simulink library "dkc"  (R2021b)
settings: Solver=VariableStepAuto  StartTime=0.0  StopTime=10.0  RelTol=1e-3
undefined symbols (not defined in the file or in its folder): ENUM_ANTITHEFT_ALARM, ENUM_ANTITHEFT_ARM, ENUM_ANTITHEFT_DISARM, ENUM_ANTITHEFT_WAIT, ENUM_BTCONNSTA_CONNECTED, ENUM_BTConnSta_CONNECTED, ENUM_BTCONNSTA_DISCONNECTED, ENUM_DKCAuthSta_DECRYPTIONFAIL, ENUM_DKCAuthSta_NORMAL, ENUM_DKCAuthSta_TIMEERROR, ENUM_DKCPCMDHANDING_FORCELIFT, ENUM_DKCPCMDHANDING_LOCK, ENUM_DKCPCMDHANDING_LOCKTGATEFAIL, ENUM_DKCPCMDHANDING_OVER, ENUM_DKCPCMDHANDING_TGATEHANDLE, ENUM_DKCPCMDHANDING_UNLOCK, ENUM_DkeyShowIVI_DEFAULT, ENUM_DkeyShowIVI_INVALID, ENUM_DkeyShowIVI_NFCGREEN, ENUM_DkeyShowIVI_NFCRED, ENUM_GEARACTUALPOSN_N, ENUM_GEARACTUALPOSN_P, ENUM_KEYMISSSTA_DEFAULT, ENUM_KEYMISSSTA_KEYMISS, ENUM_KEYMODE_DAFAULT, ENUM_KEYMODE_INVALID, ENUM_KEYMODE_NFC, ENUM_KEYMODE_UIDBLE, ENUM_KEYMODE_UIDUWB, ENUM_KEYTYPE_NFC, ENUM_KEYTYPE_NOREQ, ENUM_KEYTYPE_UID, ENUM_PCMDTOBCM_DEFAULT, ENUM_PCMDTOBCM_FORCELIFT, ENUM_PCMDTOBCM_LOCK, ENUM_PCMDTOBCM_LOCKTGATEFAIL, ENUM_PCMDTOBCM_NFCCOMMAND, ENUM_PCMDTOBCM_REMOTETGATE, ENUM_PCMDTOBCM_TGATEHANDLE, ENUM_PCMDTOBCM_UNLOCK, ENUM_PCMDTOBCM_UWBLOCK, ENUM_PCMDTOBCM_UWBUNLOCK, ENUM_PDKEYPTGRAW_INTOZONE, ENUM_PDKEYPTGRAW_OUTZONE, ENUM_PDKEYPTGRAW_UNAVALIABLE, ENUM_PDKEYRAWLULOCK_INLOCK, ENUM_PDKEYRAWLULOCK_INUNLOCK, ENUM_PDKEYRAWLULOCK_UNAVALIABLE, ENUM_PDKEYRAWPS_INPS, ENUM_PDKEYRAWPS_OUTPS, ENUM_PDKEYRAWPS_UNAVALIABLE, ENUM_PDKEYSPTGRAW_INTOZONE, ENUM_PDKEYSPTGRAW_OUTZONE, ENUM_PDKEYSPTGRAW_UNAVALIABLE, ENUM_PDKEYWELCOMERAW_INTOZONE, ENUM_PDKEYWELCOMERAW_UNAVALIABLE, ENUM_POWERSTA_OFF, ENUM_POWERSTA_OFFA, ENUM_POWERSTA_OFFC, ENUM_POWERSTA_ON ... (+79)
libraries: simulink x99, hcu_lib x6
(part 3 of 4)

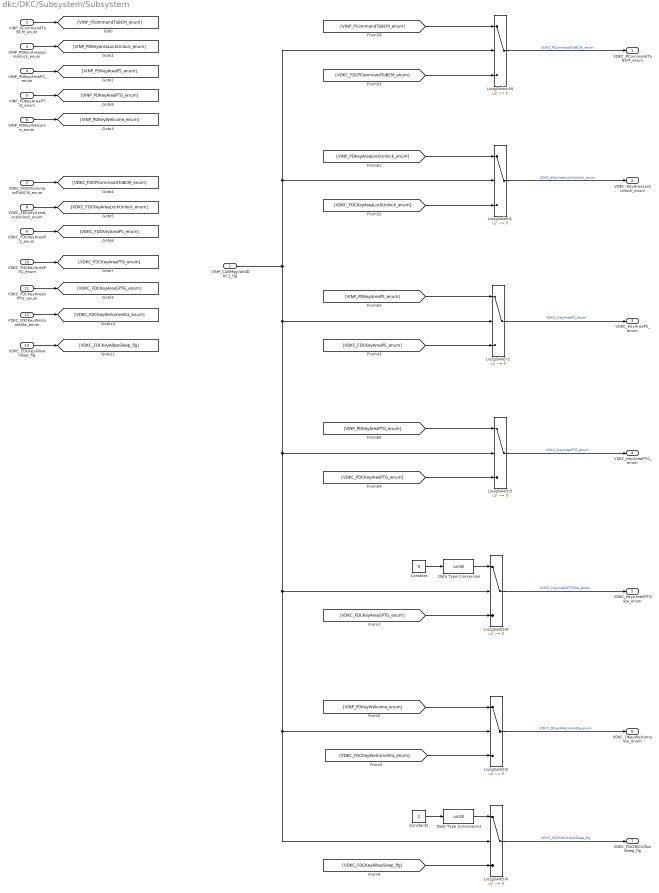
== system dkc/DKC/Subsystem/Subsystem ==
  VINP_CANMsgValidDKC1_flg : Inport
  VINP_PCommandToBCM_enum : Inport  Port=2
  VINP_PDKeyAreaLockUnlock_enum : Inport  Port=3
  VINP_PDKeyAreaPS_enum : Inport  Port=4
  VINP_PDKeyAreaPTG_enum : Inport  Port=5
  VINP_PDKeyWelcome_enum : Inport  Port=6
  VDKC_FDCPCommandToBCM_enum : Inport  Port=7
  VDKC_FDCKeyAreaLockUnlock_enum : Inport  Port=8
  VDKC_FDCKeyAreaPS_enum : Inport  Port=9
  VDKC_FDCKeyAreaPTG_enum : Inport  Port=10
  VDKC_FDCKeyAreaSPTG_enum : Inport  Port=11
  VDKC_FDCKeyWelcomeSta_enum : Inport  Port=12
  VDKC_FDCKeyAllowSleep_flg : Inport  Port=13
  Constant : Constant  Value=0
  Constant1 : Constant
  Data Type Conversion : DataTypeConversion  OutDataTypeStr=uint8
  Data Type Conversion1 : DataTypeConversion  OutDataTypeStr=uint8
  LiuzgSwitch{1..6,16} (7 alike) : Switch  Criteria=u2 ~= 0
      settings: AttributesFormatString=<%<Criteria>>
  VDKC_PCommandToBCM_enum : Outport
  VDKC_KeyAreaLockUnlock_enum : Outport  Port=2
  VDKC_KeyAreaPS_enum : Outport  Port=3
  VDKC_KeyAreaPTG_enum : Outport  Port=4
  VDKC_KeyAreaSPTGSta_enum : Outport  Port=5
  VDKC_DKeyWelcomeSta_enum : Outport  Port=6
  VDKC_FDCDKCAllowSleep_flg : Outport  Port=7
  wires:
  LiuzgSwitch6/1 -> VDKC_FDCDKCAllowSleep_flg/1  "VDKC_FDCDKCAllowSleep_flg"
  [VDKC_FDCKeyAllowSleep_flg] -> LiuzgSwitch6/3
  Data Type Conversion1/1 -> LiuzgSwitch6/1
  Constant1/1 -> Data Type Conversion1/1
  VDKC_FDCKeyAllowSleep_flg/1 -> [VDKC_FDCKeyAllowSleep_flg]
  Constant/1 -> Data Type Conversion/1
  Data Type Conversion/1 -> LiuzgSwitch4/1
  [VDKC_FDCKeyAreaSPTG_enum] -> LiuzgSwitch4/3
  VDKC_FDCKeyAreaSPTG_enum/1 -> [VDKC_FDCKeyAreaSPTG_enum]
  [VINP_PDKeyAreaPTG_enum] -> LiuzgSwitch3/1
  LiuzgSwitch4/1 -> VDKC_KeyAreaSPTGSta_enum/1  "VDKC_KeyAreaSPTGSta_enum"
  VINP_CANMsgValidDKC1_flg/1 -> LiuzgSwitch1/2, LiuzgSwitch16/2, LiuzgSwitch3/2, LiuzgSwitch6/2, LiuzgSwitch5/2, LiuzgSwitch4/2, LiuzgSwitch2/2
  VINP_PDKeyAreaPTG_enum/1 -> [VINP_PDKeyAreaPTG_enum]
  [VDKC_FDCKeyAreaPS_enum] -> LiuzgSwitch2/3
  [VDKC_FDCKeyAreaPTG_enum] -> LiuzgSwitch3/3
  LiuzgSwitch2/1 -> VDKC_KeyAreaPS_enum/1  "VDKC_KeyAreaPS_enum"
  [VINP_PCommandToBCM_enum] -> LiuzgSwitch16/1
  LiuzgSwitch3/1 -> VDKC_KeyAreaPTG_enum/1  "VDKC_KeyAreaPTG_enum"
  [VINP_PDKeyAreaLockUnlock_enum] -> LiuzgSwitch1/1
  [VDKC_FDCPCommandToBCM_enum] -> LiuzgSwitch16/3
  [VDKC_FDCKeyAreaLockUnlock_enum] -> LiuzgSwitch1/3
  [VINP_PDKeyAreaPS_enum] -> LiuzgSwitch2/1
  LiuzgSwitch16/1 -> VDKC_PCommandToBCM_enum/1  "VDKC_PCommandToBCM_enum"
  LiuzgSwitch1/1 -> VDKC_KeyAreaLockUnlock_enum/1  "VDKC_KeyAreaLockUnlock_enum"
  VINP_PCommandToBCM_enum/1 -> [VINP_PCommandToBCM_enum]
  VINP_PDKeyAreaLockUnlock_enum/1 -> [VINP_PDKeyAreaLockUnlock_enum]
  VINP_PDKeyAreaPS_enum/1 -> [VINP_PDKeyAreaPS_enum]
  VDKC_FDCKeyAreaPTG_enum/1 -> [VDKC_FDCKeyAreaPTG_enum]
  VDKC_FDCKeyAreaPS_enum/1 -> [VDKC_FDCKeyAreaPS_enum]
  VDKC_FDCKeyAreaLockUnlock_enum/1 -> [VDKC_FDCKeyAreaLockUnlock_enum]
  VDKC_FDCPCommandToBCM_enum/1 -> [VDKC_FDCPCommandToBCM_enum]
  LiuzgSwitch5/1 -> VDKC_DKeyWelcomeSta_enum/1  "VDKC_DKeyWelcomeSta_enum"
  VINP_PDKeyWelcome_enum/1 -> [VINP_PDKeyWelcome_enum]
  [VINP_PDKeyWelcome_enum] -> LiuzgSwitch5/1
  VDKC_FDCKeyWelcomeSta_enum/1 -> [VDKC_FDCKeyWelcomeSta_enum]
  [VDKC_FDCKeyWelcomeSta_enum] -> LiuzgSwitch5/3

== system dkc/DKC/Subsystem/Triggered Subsystem ==
  Trigger : TriggerPort  TriggerType=function-call  VariantControl=(inherit)
  RollingCounter : Subsystem  mask{CounterMAX=4294967295}
      mask help: MeasumentTrigerEvent
      mask Display: fprintf('RollingCounter');
  DKCTimeSN : Outport
  wires:
  RollingCounter/1(out) -> DKCTimeSN/1

== system dkc/DKC/Subsystem/DKC_Handler/SR_Latch1 ==
  set : Inport
  reset : Inport  Port=2
  Data Type Conversion : DataTypeConversion  OutDataTypeStr=boolean
  Logical Operator : Logic  AllPortsSameDT=off  OutDataTypeStr=boolean
  Logical Operator1 : Logic  Operator=NOT  AllPortsSameDT=off  OutDataTypeStr=boolean
  Switch1 : Switch  Criteria=u2 ~= 0  Threshold=0.5
      settings: AttributesFormatString=<Criteria=%<Criteria>>
  Switch2 : Switch  Criteria=u2 ~= 0  Threshold=0.5
      settings: AttributesFormatString=<Criteria=%<Criteria>>
  Unit Delay : UnitDelay  SampleTime=-1  HasFrameUpgradeWarning=on
  latched : Outport
  wires:
  Logical Operator1/1 -> Switch2/1, Logical Operator/2
  Logical Operator/1 -> Switch1/2
  Switch2/1 -> Switch1/3
  Unit Delay/1 -> Switch2/3
  reset/1 -> Logical Operator1/1, Switch2/2
  set/1 -> Logical Operator/1, Switch1/1
  Switch1/1 -> Data Type Conversion/1
  Data Type Conversion/1 -> latched/1, Unit Delay/1

== system dkc/DKC/Subsystem/DKC_Handler/SR_Latch10 ==
  set : Inport
  reset : Inport  Port=2
  Data Type Conversion : DataTypeConversion  OutDataTypeStr=boolean
  Logical Operator : Logic  AllPortsSameDT=off  OutDataTypeStr=boolean
  Logical Operator1 : Logic  Operator=NOT  AllPortsSameDT=off  OutDataTypeStr=boolean
  Switch1 : Switch  Criteria=u2 ~= 0  Threshold=0.5
      settings: AttributesFormatString=<Criteria=%<Criteria>>
  Switch2 : Switch  Criteria=u2 ~= 0  Threshold=0.5
      settings: AttributesFormatString=<Criteria=%<Criteria>>
  Unit Delay : UnitDelay  SampleTime=-1  HasFrameUpgradeWarning=on
  latched : Outport
  wires:
  Logical Operator1/1 -> Switch2/1, Logical Operator/2
  Logical Operator/1 -> Switch1/2
  Switch2/1 -> Switch1/3
  Unit Delay/1 -> Switch2/3
  reset/1 -> Logical Operator1/1, Switch2/2
  set/1 -> Logical Operator/1, Switch1/1
  Switch1/1 -> Data Type Conversion/1
  Data Type Conversion/1 -> latched/1, Unit Delay/1

== system dkc/DKC/Subsystem/DKC_Handler/SR_Latch11 ==
  set : Inport
  reset : Inport  Port=2
  Data Type Conversion : DataTypeConversion  OutDataTypeStr=boolean
  Logical Operator : Logic  AllPortsSameDT=off  OutDataTypeStr=boolean
  Logical Operator1 : Logic  Operator=NOT  AllPortsSameDT=off  OutDataTypeStr=boolean
  Switch1 : Switch  Criteria=u2 ~= 0  Threshold=0.5
      settings: AttributesFormatString=<Criteria=%<Criteria>>
  Switch2 : Switch  Criteria=u2 ~= 0  Threshold=0.5
      settings: AttributesFormatString=<Criteria=%<Criteria>>
  Unit Delay : UnitDelay  SampleTime=-1  HasFrameUpgradeWarning=on
  latched : Outport
  wires:
  Data Type Conversion/1 -> Unit Delay/1, latched/1
  Switch1/1 -> Data Type Conversion/1
  set/1 -> Switch1/1, Logical Operator/1
  reset/1 -> Switch2/2, Logical Operator1/1
  Unit Delay/1 -> Switch2/3
  Switch2/1 -> Switch1/3
  Logical Operator/1 -> Switch1/2
  Logical Operator1/1 -> Logical Operator/2, Switch2/1

== system dkc/DKC/Subsystem/DKC_Handler/SR_Latch12 ==
  set : Inport
  reset : Inport  Port=2
  Data Type Conversion : DataTypeConversion  OutDataTypeStr=boolean
  Logical Operator : Logic  AllPortsSameDT=off  OutDataTypeStr=boolean
  Logical Operator1 : Logic  Operator=NOT  AllPortsSameDT=off  OutDataTypeStr=boolean
  Switch1 : Switch  Criteria=u2 ~= 0  Threshold=0.5
      settings: AttributesFormatString=<Criteria=%<Criteria>>
  Switch2 : Switch  Criteria=u2 ~= 0  Threshold=0.5
      settings: AttributesFormatString=<Criteria=%<Criteria>>
  Unit Delay : UnitDelay  SampleTime=-1  HasFrameUpgradeWarning=on
  latched : Outport
  wires:
  Data Type Conversion/1 -> Unit Delay/1, latched/1
  Switch1/1 -> Data Type Conversion/1
  set/1 -> Switch1/1, Logical Operator/1
  reset/1 -> Switch2/2, Logical Operator1/1
  Unit Delay/1 -> Switch2/3
  Switch2/1 -> Switch1/3
  Logical Operator/1 -> Switch1/2
  Logical Operator1/1 -> Logical Operator/2, Switch2/1

== system dkc/DKC/Subsystem/DKC_Handler/SR_Latch13 ==
  set : Inport
  reset : Inport  Port=2
  Data Type Conversion : DataTypeConversion  OutDataTypeStr=boolean
  Logical Operator : Logic  AllPortsSameDT=off  OutDataTypeStr=boolean
  Logical Operator1 : Logic  Operator=NOT  AllPortsSameDT=off  OutDataTypeStr=boolean
  Switch1 : Switch  Criteria=u2 ~= 0  Threshold=0.5
      settings: AttributesFormatString=<Criteria=%<Criteria>>
  Switch2 : Switch  Criteria=u2 ~= 0  Threshold=0.5
      settings: AttributesFormatString=<Criteria=%<Criteria>>
  Unit Delay : UnitDelay  SampleTime=-1  HasFrameUpgradeWarning=on
  latched : Outport
  wires:
  Logical Operator1/1 -> Switch2/1, Logical Operator/2
  Logical Operator/1 -> Switch1/2
  Switch2/1 -> Switch1/3
  Unit Delay/1 -> Switch2/3
  reset/1 -> Logical Operator1/1, Switch2/2
  set/1 -> Logical Operator/1, Switch1/1
  Switch1/1 -> Data Type Conversion/1
  Data Type Conversion/1 -> latched/1, Unit Delay/1

== system dkc/DKC/Subsystem/DKC_Handler/SR_Latch14 ==
  set : Inport
  reset : Inport  Port=2
  Data Type Conversion : DataTypeConversion  OutDataTypeStr=boolean
  Logical Operator : Logic  AllPortsSameDT=off  OutDataTypeStr=boolean
  Logical Operator1 : Logic  Operator=NOT  AllPortsSameDT=off  OutDataTypeStr=boolean
  Switch1 : Switch  Criteria=u2 ~= 0  Threshold=0.5
      settings: AttributesFormatString=<Criteria=%<Criteria>>
  Switch2 : Switch  Criteria=u2 ~= 0  Threshold=0.5
      settings: AttributesFormatString=<Criteria=%<Criteria>>
  Unit Delay : UnitDelay  SampleTime=-1  HasFrameUpgradeWarning=on
  latched : Outport
  wires:
  Data Type Conversion/1 -> Unit Delay/1, latched/1
  Switch1/1 -> Data Type Conversion/1
  set/1 -> Switch1/1, Logical Operator/1
  reset/1 -> Switch2/2, Logical Operator1/1
  Unit Delay/1 -> Switch2/3
  Switch2/1 -> Switch1/3
  Logical Operator/1 -> Switch1/2
  Logical Operator1/1 -> Logical Operator/2, Switch2/1

== system dkc/DKC/Subsystem/DKC_Handler/SR_Latch15 ==
  set : Inport
  reset : Inport  Port=2
  Data Type Conversion : DataTypeConversion  OutDataTypeStr=boolean
  Logical Operator : Logic  AllPortsSameDT=off  OutDataTypeStr=boolean
  Logical Operator1 : Logic  Operator=NOT  AllPortsSameDT=off  OutDataTypeStr=boolean
  Switch1 : Switch  Criteria=u2 ~= 0  Threshold=0.5
      settings: AttributesFormatString=<Criteria=%<Criteria>>
  Switch2 : Switch  Criteria=u2 ~= 0  Threshold=0.5
      settings: AttributesFormatString=<Criteria=%<Criteria>>
  Unit Delay : UnitDelay  SampleTime=-1  HasFrameUpgradeWarning=on
  latched : Outport
  wires:
  Logical Operator1/1 -> Switch2/1, Logical Operator/2
  Logical Operator/1 -> Switch1/2
  Switch2/1 -> Switch1/3
  Unit Delay/1 -> Switch2/3
  reset/1 -> Logical Operator1/1, Switch2/2
  set/1 -> Logical Operator/1, Switch1/1
  Switch1/1 -> Data Type Conversion/1
  Data Type Conversion/1 -> latched/1, Unit Delay/1

== system dkc/DKC/Subsystem/DKC_Handler/SR_Latch16 ==
  set : Inport
  reset : Inport  Port=2
  Data Type Conversion : DataTypeConversion  OutDataTypeStr=boolean
  Logical Operator : Logic  AllPortsSameDT=off  OutDataTypeStr=boolean
  Logical Operator1 : Logic  Operator=NOT  AllPortsSameDT=off  OutDataTypeStr=boolean
  Switch1 : Switch  Criteria=u2 ~= 0  Threshold=0.5
      settings: AttributesFormatString=<Criteria=%<Criteria>>
  Switch2 : Switch  Criteria=u2 ~= 0  Threshold=0.5
      settings: AttributesFormatString=<Criteria=%<Criteria>>
  Unit Delay : UnitDelay  SampleTime=-1  HasFrameUpgradeWarning=on
  latched : Outport
  wires:
  Data Type Conversion/1 -> Unit Delay/1, latched/1
  Switch1/1 -> Data Type Conversion/1
  set/1 -> Switch1/1, Logical Operator/1
  reset/1 -> Switch2/2, Logical Operator1/1
  Unit Delay/1 -> Switch2/3
  Switch2/1 -> Switch1/3
  Logical Operator/1 -> Switch1/2
  Logical Operator1/1 -> Logical Operator/2, Switch2/1

== system dkc/DKC/Subsystem/DKC_Handler/SR_Latch17 ==
  set : Inport
  reset : Inport  Port=2
  Data Type Conversion : DataTypeConversion  OutDataTypeStr=boolean
  Logical Operator : Logic  AllPortsSameDT=off  OutDataTypeStr=boolean
  Logical Operator1 : Logic  Operator=NOT  AllPortsSameDT=off  OutDataTypeStr=boolean
  Switch1 : Switch  Criteria=u2 ~= 0  Threshold=0.5
      settings: AttributesFormatString=<Criteria=%<Criteria>>
  Switch2 : Switch  Criteria=u2 ~= 0  Threshold=0.5
      settings: AttributesFormatString=<Criteria=%<Criteria>>
  Unit Delay : UnitDelay  SampleTime=-1  HasFrameUpgradeWarning=on
  latched : Outport
  wires:
  Logical Operator1/1 -> Switch2/1, Logical Operator/2
  Logical Operator/1 -> Switch1/2
  Switch2/1 -> Switch1/3
  Unit Delay/1 -> Switch2/3
  reset/1 -> Logical Operator1/1, Switch2/2
  set/1 -> Logical Operator/1, Switch1/1
  Switch1/1 -> Data Type Conversion/1
  Data Type Conversion/1 -> latched/1, Unit Delay/1

== system dkc/DKC/Subsystem/DKC_Handler/SR_Latch18 ==
  set : Inport
  reset : Inport  Port=2
  Data Type Conversion : DataTypeConversion  OutDataTypeStr=boolean
  Logical Operator : Logic  AllPortsSameDT=off  OutDataTypeStr=boolean
  Logical Operator1 : Logic  Operator=NOT  AllPortsSameDT=off  OutDataTypeStr=boolean
  Switch1 : Switch  Criteria=u2 ~= 0  Threshold=0.5
      settings: AttributesFormatString=<Criteria=%<Criteria>>
  Switch2 : Switch  Criteria=u2 ~= 0  Threshold=0.5
      settings: AttributesFormatString=<Criteria=%<Criteria>>
  Unit Delay : UnitDelay  SampleTime=-1  HasFrameUpgradeWarning=on
  latched : Outport
  wires:
  Data Type Conversion/1 -> Unit Delay/1, latched/1
  Switch1/1 -> Data Type Conversion/1
  set/1 -> Switch1/1, Logical Operator/1
  reset/1 -> Switch2/2, Logical Operator1/1
  Unit Delay/1 -> Switch2/3
  Switch2/1 -> Switch1/3
  Logical Operator/1 -> Switch1/2
  Logical Operator1/1 -> Logical Operator/2, Switch2/1

== system dkc/DKC/Subsystem/DKC_Handler/SR_Latch19 ==
  set : Inport
  reset : Inport  Port=2
  Data Type Conversion : DataTypeConversion  OutDataTypeStr=boolean
  Logical Operator : Logic  AllPortsSameDT=off  OutDataTypeStr=boolean
  Logical Operator1 : Logic  Operator=NOT  AllPortsSameDT=off  OutDataTypeStr=boolean
  Switch1 : Switch  Criteria=u2 ~= 0  Threshold=0.5
      settings: AttributesFormatString=<Criteria=%<Criteria>>
  Switch2 : Switch  Criteria=u2 ~= 0  Threshold=0.5
      settings: AttributesFormatString=<Criteria=%<Criteria>>
  Unit Delay : UnitDelay  SampleTime=-1  HasFrameUpgradeWarning=on
  latched : Outport
  wires:
  Data Type Conversion/1 -> Unit Delay/1, latched/1
  Switch1/1 -> Data Type Conversion/1
  set/1 -> Switch1/1, Logical Operator/1
  reset/1 -> Switch2/2, Logical Operator1/1
  Unit Delay/1 -> Switch2/3
  Switch2/1 -> Switch1/3
  Logical Operator/1 -> Switch1/2
  Logical Operator1/1 -> Logical Operator/2, Switch2/1

== system dkc/DKC/Subsystem/DKC_Handler/SR_Latch2 ==
  set : Inport
  reset : Inport  Port=2
  Data Type Conversion : DataTypeConversion  OutDataTypeStr=boolean
  Logical Operator : Logic  AllPortsSameDT=off  OutDataTypeStr=boolean
  Logical Operator1 : Logic  Operator=NOT  AllPortsSameDT=off  OutDataTypeStr=boolean
  Switch1 : Switch  Criteria=u2 ~= 0  Threshold=0.5
      settings: AttributesFormatString=<Criteria=%<Criteria>>
  Switch2 : Switch  Criteria=u2 ~= 0  Threshold=0.5
      settings: AttributesFormatString=<Criteria=%<Criteria>>
  Unit Delay : UnitDelay  SampleTime=-1  HasFrameUpgradeWarning=on
  latched : Outport
  wires:
  Data Type Conversion/1 -> Unit Delay/1, latched/1
  Switch1/1 -> Data Type Conversion/1
  set/1 -> Switch1/1, Logical Operator/1
  reset/1 -> Switch2/2, Logical Operator1/1
  Unit Delay/1 -> Switch2/3
  Switch2/1 -> Switch1/3
  Logical Operator/1 -> Switch1/2
  Logical Operator1/1 -> Logical Operator/2, Switch2/1

== system dkc/DKC/Subsystem/DKC_Handler/SR_Latch20 ==
  set : Inport
  reset : Inport  Port=2
  Data Type Conversion : DataTypeConversion  OutDataTypeStr=boolean
  Logical Operator : Logic  AllPortsSameDT=off  OutDataTypeStr=boolean
  Logical Operator1 : Logic  Operator=NOT  AllPortsSameDT=off  OutDataTypeStr=boolean
  Switch1 : Switch  Criteria=u2 ~= 0  Threshold=0.5
      settings: AttributesFormatString=<Criteria=%<Criteria>>
  Switch2 : Switch  Criteria=u2 ~= 0  Threshold=0.5
      settings: AttributesFormatString=<Criteria=%<Criteria>>
  Unit Delay : UnitDelay  SampleTime=-1  HasFrameUpgradeWarning=on
  latched : Outport
  wires:
  Data Type Conversion/1 -> Unit Delay/1, latched/1
  Switch1/1 -> Data Type Conversion/1
  set/1 -> Switch1/1, Logical Operator/1
  reset/1 -> Switch2/2, Logical Operator1/1
  Unit Delay/1 -> Switch2/3
  Switch2/1 -> Switch1/3
  Logical Operator/1 -> Switch1/2
  Logical Operator1/1 -> Logical Operator/2, Switch2/1

== system dkc/DKC/Subsystem/DKC_Handler/SR_Latch4 ==
  set : Inport
  reset : Inport  Port=2
  Data Type Conversion : DataTypeConversion  OutDataTypeStr=boolean
  Logical Operator : Logic  AllPortsSameDT=off  OutDataTypeStr=boolean
  Logical Operator1 : Logic  Operator=NOT  AllPortsSameDT=off  OutDataTypeStr=boolean
  Switch1 : Switch  Criteria=u2 ~= 0  Threshold=0.5
      settings: AttributesFormatString=<Criteria=%<Criteria>>
  Switch2 : Switch  Criteria=u2 ~= 0  Threshold=0.5
      settings: AttributesFormatString=<Criteria=%<Criteria>>
  Unit Delay : UnitDelay  SampleTime=-1  HasFrameUpgradeWarning=on
  latched : Outport
  wires:
  Logical Operator1/1 -> Switch2/1, Logical Operator/2
  Logical Operator/1 -> Switch1/2
  Switch2/1 -> Switch1/3
  Unit Delay/1 -> Switch2/3
  reset/1 -> Logical Operator1/1, Switch2/2
  set/1 -> Logical Operator/1, Switch1/1
  Switch1/1 -> Data Type Conversion/1
  Data Type Conversion/1 -> latched/1, Unit Delay/1

== system dkc/DKC/Subsystem/DKC_Handler/SR_Latch5 ==
  set : Inport
  reset : Inport  Port=2
  Data Type Conversion : DataTypeConversion  OutDataTypeStr=boolean
  Logical Operator : Logic  AllPortsSameDT=off  OutDataTypeStr=boolean
  Logical Operator1 : Logic  Operator=NOT  AllPortsSameDT=off  OutDataTypeStr=boolean
  Switch1 : Switch  Criteria=u2 ~= 0  Threshold=0.5
      settings: AttributesFormatString=<Criteria=%<Criteria>>
  Switch2 : Switch  Criteria=u2 ~= 0  Threshold=0.5
      settings: AttributesFormatString=<Criteria=%<Criteria>>
  Unit Delay : UnitDelay  SampleTime=-1  HasFrameUpgradeWarning=on
  latched : Outport
  wires:
  Data Type Conversion/1 -> Unit Delay/1, latched/1
  Switch1/1 -> Data Type Conversion/1
  set/1 -> Switch1/1, Logical Operator/1
  reset/1 -> Switch2/2, Logical Operator1/1
  Unit Delay/1 -> Switch2/3
  Switch2/1 -> Switch1/3
  Logical Operator/1 -> Switch1/2
  Logical Operator1/1 -> Logical Operator/2, Switch2/1

== system dkc/DKC/Subsystem/DKC_Handler/SR_Latch6 ==
  set : Inport
  reset : Inport  Port=2
  Data Type Conversion : DataTypeConversion  OutDataTypeStr=boolean
  Logical Operator : Logic  AllPortsSameDT=off  OutDataTypeStr=boolean
  Logical Operator1 : Logic  Operator=NOT  AllPortsSameDT=off  OutDataTypeStr=boolean
  Switch1 : Switch  Criteria=u2 ~= 0  Threshold=0.5
      settings: AttributesFormatString=<Criteria=%<Criteria>>
  Switch2 : Switch  Criteria=u2 ~= 0  Threshold=0.5
      settings: AttributesFormatString=<Criteria=%<Criteria>>
  Unit Delay : UnitDelay  SampleTime=-1  HasFrameUpgradeWarning=on
  latched : Outport
  wires:
  Logical Operator1/1 -> Switch2/1, Logical Operator/2
  Logical Operator/1 -> Switch1/2
  Switch2/1 -> Switch1/3
  Unit Delay/1 -> Switch2/3
  reset/1 -> Logical Operator1/1, Switch2/2
  set/1 -> Logical Operator/1, Switch1/1
  Switch1/1 -> Data Type Conversion/1
  Data Type Conversion/1 -> latched/1, Unit Delay/1

== system dkc/DKC/Subsystem/DKC_Handler/SR_Latch8 ==
  set : Inport
  reset : Inport  Port=2
  Data Type Conversion : DataTypeConversion  OutDataTypeStr=boolean
  Logical Operator : Logic  AllPortsSameDT=off  OutDataTypeStr=boolean
  Logical Operator1 : Logic  Operator=NOT  AllPortsSameDT=off  OutDataTypeStr=boolean
  Switch1 : Switch  Criteria=u2 ~= 0  Threshold=0.5
      settings: AttributesFormatString=<Criteria=%<Criteria>>
  Switch2 : Switch  Criteria=u2 ~= 0  Threshold=0.5
      settings: AttributesFormatString=<Criteria=%<Criteria>>
  Unit Delay : UnitDelay  SampleTime=-1  HasFrameUpgradeWarning=on
  latched : Outport
  wires:
  Logical Operator1/1 -> Switch2/1, Logical Operator/2
  Logical Operator/1 -> Switch1/2
  Switch2/1 -> Switch1/3
  Unit Delay/1 -> Switch2/3
  reset/1 -> Logical Operator1/1, Switch2/2
  set/1 -> Logical Operator/1, Switch1/1
  Switch1/1 -> Data Type Conversion/1
  Data Type Conversion/1 -> latched/1, Unit Delay/1

== system dkc/DKC/Subsystem/DKC_Handler/SR_Latch9 ==
  set : Inport
  reset : Inport  Port=2
  Data Type Conversion : DataTypeConversion  OutDataTypeStr=boolean
  Logical Operator : Logic  AllPortsSameDT=off  OutDataTypeStr=boolean
  Logical Operator1 : Logic  Operator=NOT  AllPortsSameDT=off  OutDataTypeStr=boolean
  Switch1 : Switch  Criteria=u2 ~= 0  Threshold=0.5
      settings: AttributesFormatString=<Criteria=%<Criteria>>
  Switch2 : Switch  Criteria=u2 ~= 0  Threshold=0.5
      settings: AttributesFormatString=<Criteria=%<Criteria>>
  Unit Delay : UnitDelay  SampleTime=-1  HasFrameUpgradeWarning=on
  latched : Outport
  wires:
  Data Type Conversion/1 -> Unit Delay/1, latched/1
  Switch1/1 -> Data Type Conversion/1
  set/1 -> Switch1/1, Logical Operator/1
  reset/1 -> Switch2/2, Logical Operator1/1
  Unit Delay/1 -> Switch2/3
  Switch2/1 -> Switch1/3
  Logical Operator/1 -> Switch1/2
  Logical Operator1/1 -> Logical Operator/2, Switch2/1

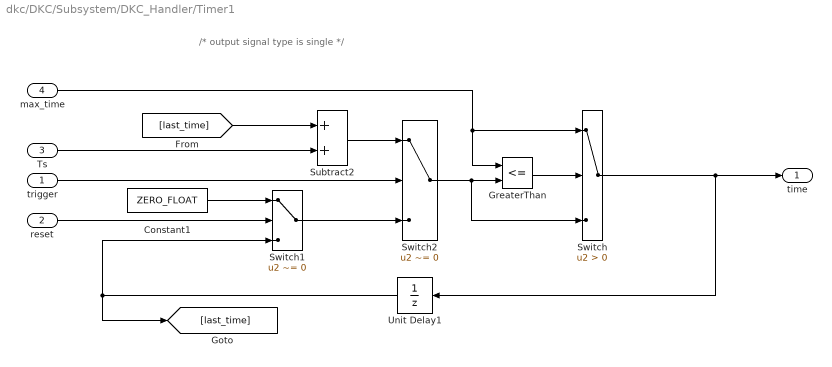
== system dkc/DKC/Subsystem/DKC_Handler/Timer1 ==
  note: /* output signal type is single */
  trigger : Inport
  reset : Inport  Port=2
  Ts : Inport  Port=3
  max_time : Inport  Port=4
  Constant1 : Constant  Value=ZERO_FLOAT  OutDataTypeStr=single
  GreaterThan : RelationalOperator  Operator=<=  OutDataTypeStr=boolean  RndMeth=Simplest
  Subtract2 : Sum
  Switch : Switch  Criteria=u2 > Threshold
  Switch1 : Switch  Criteria=u2 ~= 0
      settings: AttributesFormatString=<%<Criteria>>
  Switch2 : Switch  Criteria=u2 ~= 0
      settings: AttributesFormatString=<%<Criteria>>
  Unit Delay1 : UnitDelay  SampleTime=-1  HasFrameUpgradeWarning=on
      settings: AttributesFormatString=<initial = %<X0>>
  time : Outport
  wires:
  [last_time] -> Subtract2/1
  max_time/1 -> Switch/1, GreaterThan/1
  Unit Delay1/1 -> [last_time], Switch1/3
  Switch/1 -> time/1, Unit Delay1/1
  Switch2/1 -> Switch/3, GreaterThan/2
  Ts/1 -> Subtract2/2
  Switch1/1 -> Switch2/3
  Constant1/1 -> Switch1/1
  reset/1 -> Switch1/2
  trigger/1 -> Switch2/2
  Subtract2/1 -> Switch2/1
  GreaterThan/1 -> Switch/2

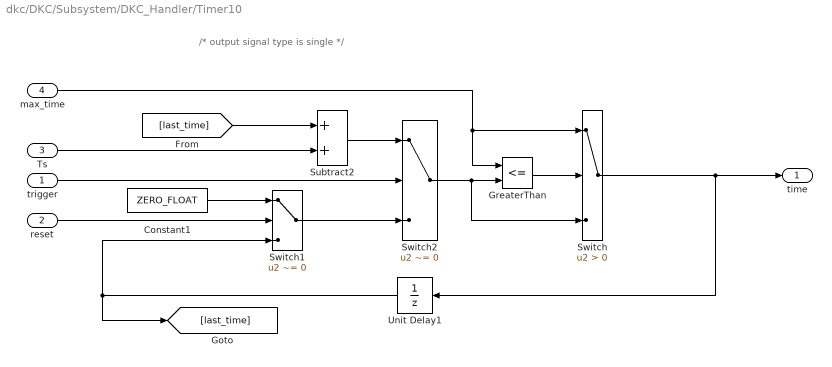
== system dkc/DKC/Subsystem/DKC_Handler/Timer10 ==
  note: /* output signal type is single */
  trigger : Inport
  reset : Inport  Port=2
  Ts : Inport  Port=3
  max_time : Inport  Port=4
  Constant1 : Constant  Value=ZERO_FLOAT  OutDataTypeStr=single
  GreaterThan : RelationalOperator  Operator=<=  OutDataTypeStr=boolean  RndMeth=Simplest
  Subtract2 : Sum
  Switch : Switch  Criteria=u2 > Threshold
  Switch1 : Switch  Criteria=u2 ~= 0
      settings: AttributesFormatString=<%<Criteria>>
  Switch2 : Switch  Criteria=u2 ~= 0
      settings: AttributesFormatString=<%<Criteria>>
  Unit Delay1 : UnitDelay  SampleTime=-1  HasFrameUpgradeWarning=on
      settings: AttributesFormatString=<initial = %<X0>>
  time : Outport
  wires:
  GreaterThan/1 -> Switch/2
  Subtract2/1 -> Switch2/1
  trigger/1 -> Switch2/2
  reset/1 -> Switch1/2
  Constant1/1 -> Switch1/1
  Switch1/1 -> Switch2/3
  Ts/1 -> Subtract2/2
  Switch2/1 -> GreaterThan/2, Switch/3
  Switch/1 -> Unit Delay1/1, time/1
  Unit Delay1/1 -> Switch1/3, [last_time]
  max_time/1 -> GreaterThan/1, Switch/1
  [last_time] -> Subtract2/1

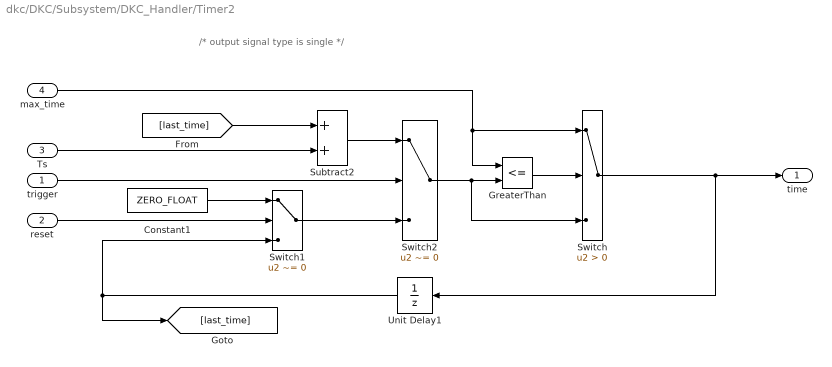
== system dkc/DKC/Subsystem/DKC_Handler/Timer2 ==
  note: /* output signal type is single */
  trigger : Inport
  reset : Inport  Port=2
  Ts : Inport  Port=3
  max_time : Inport  Port=4
  Constant1 : Constant  Value=ZERO_FLOAT  OutDataTypeStr=single
  GreaterThan : RelationalOperator  Operator=<=  OutDataTypeStr=boolean  RndMeth=Simplest
  Subtract2 : Sum
  Switch : Switch  Criteria=u2 > Threshold
  Switch1 : Switch  Criteria=u2 ~= 0
      settings: AttributesFormatString=<%<Criteria>>
  Switch2 : Switch  Criteria=u2 ~= 0
      settings: AttributesFormatString=<%<Criteria>>
  Unit Delay1 : UnitDelay  SampleTime=-1  HasFrameUpgradeWarning=on
      settings: AttributesFormatString=<initial = %<X0>>
  time : Outport
  wires:
  [last_time] -> Subtract2/1
  max_time/1 -> Switch/1, GreaterThan/1
  Unit Delay1/1 -> [last_time], Switch1/3
  Switch/1 -> time/1, Unit Delay1/1
  Switch2/1 -> Switch/3, GreaterThan/2
  Ts/1 -> Subtract2/2
  Switch1/1 -> Switch2/3
  Constant1/1 -> Switch1/1
  reset/1 -> Switch1/2
  trigger/1 -> Switch2/2
  Subtract2/1 -> Switch2/1
  GreaterThan/1 -> Switch/2

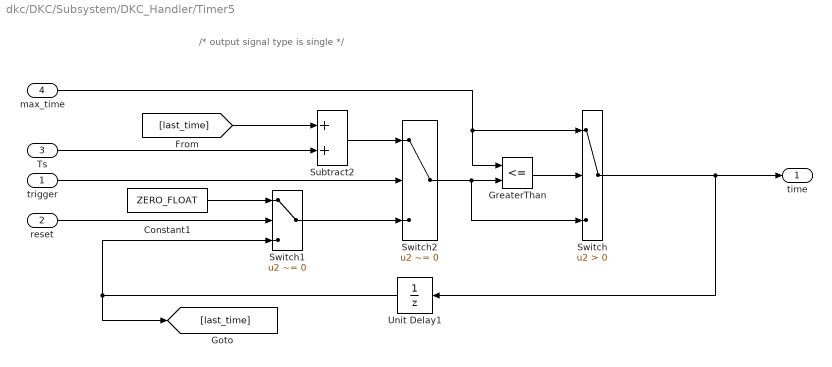
== system dkc/DKC/Subsystem/DKC_Handler/Timer5 ==
  note: /* output signal type is single */
  trigger : Inport
  reset : Inport  Port=2
  Ts : Inport  Port=3
  max_time : Inport  Port=4
  Constant1 : Constant  Value=ZERO_FLOAT  OutDataTypeStr=single
  GreaterThan : RelationalOperator  Operator=<=  OutDataTypeStr=boolean  RndMeth=Simplest
  Subtract2 : Sum
  Switch : Switch  Criteria=u2 > Threshold
  Switch1 : Switch  Criteria=u2 ~= 0
      settings: AttributesFormatString=<%<Criteria>>
  Switch2 : Switch  Criteria=u2 ~= 0
      settings: AttributesFormatString=<%<Criteria>>
  Unit Delay1 : UnitDelay  SampleTime=-1  HasFrameUpgradeWarning=on
      settings: AttributesFormatString=<initial = %<X0>>
  time : Outport
  wires:
  GreaterThan/1 -> Switch/2
  Subtract2/1 -> Switch2/1
  trigger/1 -> Switch2/2
  reset/1 -> Switch1/2
  Constant1/1 -> Switch1/1
  Switch1/1 -> Switch2/3
  Ts/1 -> Subtract2/2
  Switch2/1 -> GreaterThan/2, Switch/3
  Switch/1 -> Unit Delay1/1, time/1
  Unit Delay1/1 -> Switch1/3, [last_time]
  max_time/1 -> GreaterThan/1, Switch/1
  [last_time] -> Subtract2/1

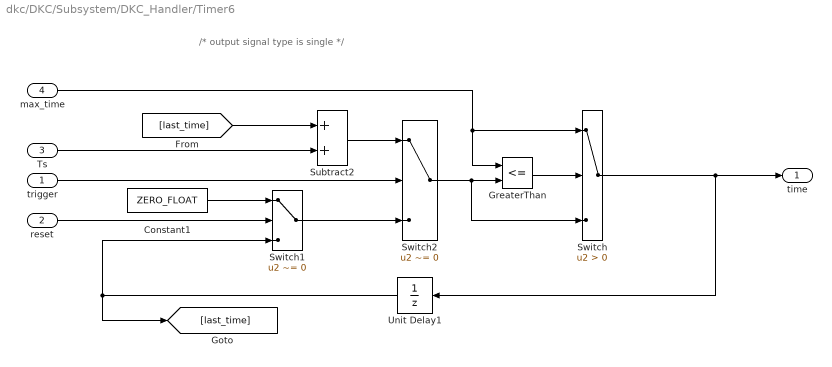
== system dkc/DKC/Subsystem/DKC_Handler/Timer6 ==
  note: /* output signal type is single */
  trigger : Inport
  reset : Inport  Port=2
  Ts : Inport  Port=3
  max_time : Inport  Port=4
  Constant1 : Constant  Value=ZERO_FLOAT  OutDataTypeStr=single
  GreaterThan : RelationalOperator  Operator=<=  OutDataTypeStr=boolean  RndMeth=Simplest
  Subtract2 : Sum
  Switch : Switch  Criteria=u2 > Threshold
  Switch1 : Switch  Criteria=u2 ~= 0
      settings: AttributesFormatString=<%<Criteria>>
  Switch2 : Switch  Criteria=u2 ~= 0
      settings: AttributesFormatString=<%<Criteria>>
  Unit Delay1 : UnitDelay  SampleTime=-1  HasFrameUpgradeWarning=on
      settings: AttributesFormatString=<initial = %<X0>>
  time : Outport
  wires:
  [last_time] -> Subtract2/1
  max_time/1 -> Switch/1, GreaterThan/1
  Unit Delay1/1 -> [last_time], Switch1/3
  Switch/1 -> time/1, Unit Delay1/1
  Switch2/1 -> Switch/3, GreaterThan/2
  Ts/1 -> Subtract2/2
  Switch1/1 -> Switch2/3
  Constant1/1 -> Switch1/1
  reset/1 -> Switch1/2
  trigger/1 -> Switch2/2
  Subtract2/1 -> Switch2/1
  GreaterThan/1 -> Switch/2

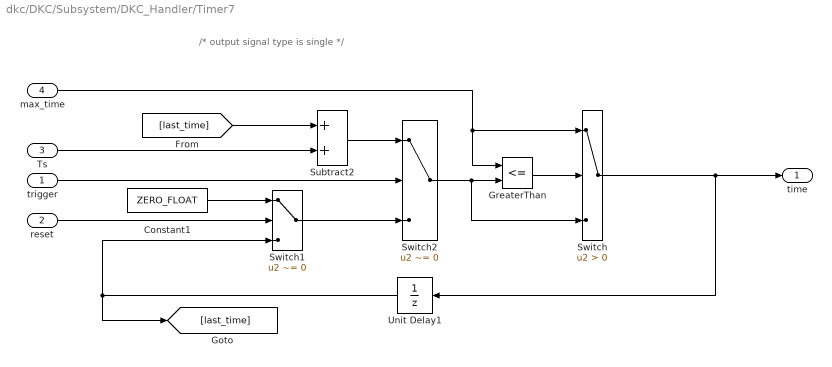
== system dkc/DKC/Subsystem/DKC_Handler/Timer7 ==
  note: /* output signal type is single */
  trigger : Inport
  reset : Inport  Port=2
  Ts : Inport  Port=3
  max_time : Inport  Port=4
  Constant1 : Constant  Value=ZERO_FLOAT  OutDataTypeStr=single
  GreaterThan : RelationalOperator  Operator=<=  OutDataTypeStr=boolean  RndMeth=Simplest
  Subtract2 : Sum
  Switch : Switch  Criteria=u2 > Threshold
  Switch1 : Switch  Criteria=u2 ~= 0
      settings: AttributesFormatString=<%<Criteria>>
  Switch2 : Switch  Criteria=u2 ~= 0
      settings: AttributesFormatString=<%<Criteria>>
  Unit Delay1 : UnitDelay  SampleTime=-1  HasFrameUpgradeWarning=on
      settings: AttributesFormatString=<initial = %<X0>>
  time : Outport
  wires:
  [last_time] -> Subtract2/1
  max_time/1 -> Switch/1, GreaterThan/1
  Unit Delay1/1 -> [last_time], Switch1/3
  Switch/1 -> time/1, Unit Delay1/1
  Switch2/1 -> Switch/3, GreaterThan/2
  Ts/1 -> Subtract2/2
  Switch1/1 -> Switch2/3
  Constant1/1 -> Switch1/1
  reset/1 -> Switch1/2
  trigger/1 -> Switch2/2
  Subtract2/1 -> Switch2/1
  GreaterThan/1 -> Switch/2

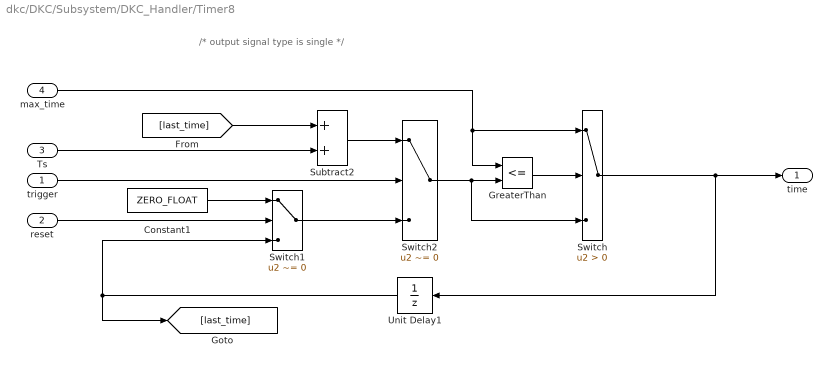
== system dkc/DKC/Subsystem/DKC_Handler/Timer8 ==
  note: /* output signal type is single */
  trigger : Inport
  reset : Inport  Port=2
  Ts : Inport  Port=3
  max_time : Inport  Port=4
  Constant1 : Constant  Value=ZERO_FLOAT  OutDataTypeStr=single
  GreaterThan : RelationalOperator  Operator=<=  OutDataTypeStr=boolean  RndMeth=Simplest
  Subtract2 : Sum
  Switch : Switch  Criteria=u2 > Threshold
  Switch1 : Switch  Criteria=u2 ~= 0
      settings: AttributesFormatString=<%<Criteria>>
  Switch2 : Switch  Criteria=u2 ~= 0
      settings: AttributesFormatString=<%<Criteria>>
  Unit Delay1 : UnitDelay  SampleTime=-1  HasFrameUpgradeWarning=on
      settings: AttributesFormatString=<initial = %<X0>>
  time : Outport
  wires:
  GreaterThan/1 -> Switch/2
  Subtract2/1 -> Switch2/1
  trigger/1 -> Switch2/2
  reset/1 -> Switch1/2
  Constant1/1 -> Switch1/1
  Switch1/1 -> Switch2/3
  Ts/1 -> Subtract2/2
  Switch2/1 -> GreaterThan/2, Switch/3
  Switch/1 -> Unit Delay1/1, time/1
  Unit Delay1/1 -> Switch1/3, [last_time]
  max_time/1 -> GreaterThan/1, Switch/1
  [last_time] -> Subtract2/1

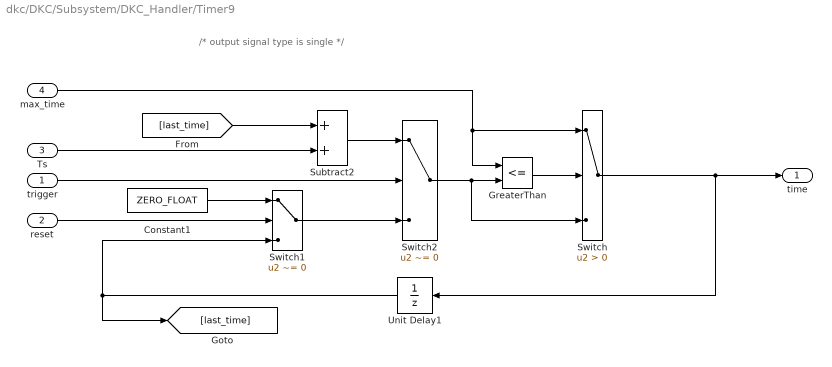
== system dkc/DKC/Subsystem/DKC_Handler/Timer9 ==
  note: /* output signal type is single */
  trigger : Inport
  reset : Inport  Port=2
  Ts : Inport  Port=3
  max_time : Inport  Port=4
  Constant1 : Constant  Value=ZERO_FLOAT  OutDataTypeStr=single
  GreaterThan : RelationalOperator  Operator=<=  OutDataTypeStr=boolean  RndMeth=Simplest
  Subtract2 : Sum
  Switch : Switch  Criteria=u2 > Threshold
  Switch1 : Switch  Criteria=u2 ~= 0
      settings: AttributesFormatString=<%<Criteria>>
  Switch2 : Switch  Criteria=u2 ~= 0
      settings: AttributesFormatString=<%<Criteria>>
  Unit Delay1 : UnitDelay  SampleTime=-1  HasFrameUpgradeWarning=on
      settings: AttributesFormatString=<initial = %<X0>>
  time : Outport
  wires:
  [last_time] -> Subtract2/1
  max_time/1 -> Switch/1, GreaterThan/1
  Unit Delay1/1 -> [last_time], Switch1/3
  Switch/1 -> time/1, Unit Delay1/1
  Switch2/1 -> Switch/3, GreaterThan/2
  Ts/1 -> Subtract2/2
  Switch1/1 -> Switch2/3
  Constant1/1 -> Switch1/1
  reset/1 -> Switch1/2
  trigger/1 -> Switch2/2
  Subtract2/1 -> Switch2/1
  GreaterThan/1 -> Switch/2

== system dkc/DKC/Subsystem/Triggered Subsystem/RollingCounter ==
  Add2 : Sum
  Constant1 : Constant  Value=ONE_INT
  Constant65 : Constant  Value=CounterMAX
  Constant67 : Constant  Value=ONE_INT
  Data Type Conversion{,1..3} (4 alike) : DataTypeConversion  OutDataTypeStr=uint32
  Equal34 : RelationalOperator  OutDataTypeStr=boolean  RndMeth=Simplest
  Switch5 : Switch  Criteria=u2 > Threshold
  Unit Delay5 : UnitDelay  SampleTime=-1  HasFrameUpgradeWarning=on
  out : Outport
  wires:
  Data Type Conversion3/1 -> Switch5/1
  Data Type Conversion2/1 -> Add2/1
  Switch5/1 -> Data Type Conversion1/1, Unit Delay5/1
  Equal34/1 -> Switch5/2
  Constant1/1 -> Data Type Conversion3/1
  Add2/1 -> Switch5/3
  Constant67/1 -> Data Type Conversion2/1
  Unit Delay5/1 -> Add2/2, Equal34/1
  Data Type Conversion/1 -> Equal34/2
  Constant65/1 -> Data Type Conversion/1
  Data Type Conversion1/1 -> out/1

== stateflow chart dkc/DKC/Subsystem/DKC_Handler/UWB_PCMD_Chart ==
  state UWB
    state UnavToUnLockReqUnlock_Cmd_Delay
      (default) -> (junction 197) : {
          |  VDKC_CmdDelayTime_s = 0;
          |  VDKC_CmdDelayDone_flg = FALSE;
          | }
      UnavToUnLockReqUnlock_Cmd_Delay -> (junction 197) [order 1]
      (junction 197) -> (junction 198) [order 1] : [ VDKC_CmdDelayTime_s > KDKC_LockCmdDelayTime_s]
      (junction 197) -> (junction 199) [order 2]
      (junction 198) -> (junction 203) : {
          |  VDKC_CmdDelayDone_flg = TRUE;
          | }
      (junction 199) -> (junction 200) [order 1] : [ VDKC_PCmdFallingEdge_flg == TRUE]
      (junction 199) -> (junction 201) [order 2] : {
          |  VDKC_CmdDelayTime_s += task_time_s;
          | }
      (junction 200) -> (junction 202) : {
          |  VDKC_CmdDelayDone_flg = TRUE;
          | }
      (junction 202) -> (junction 201)
      (junction 203) -> (junction 202)
    state RSSILock_Cmd_Delay
      (default) -> (junction 138) : {
          |  VDKC_CmdDelayTime_s = 0;
          |  VDKC_CmdDelayDone_flg = FALSE;
          | }
      RSSILock_Cmd_Delay -> (junction 138) [order 1]
      (junction 138) -> (junction 139) [order 1] : [ VDKC_CmdDelayTime_s > KDKC_LockCmdDelayTime_s]
      (junction 138) -> (junction 140) [order 2]
      (junction 139) -> (junction 144) : {
          |  VDKC_CmdDelayDone_flg = TRUE;
          | }
      (junction 140) -> (junction 141) [order 1] : [ VDKC_PCmdFallingEdge_flg == TRUE]
      (junction 140) -> (junction 142) [order 2] : {
          |  VDKC_CmdDelayTime_s += task_time_s;
          | }
      (junction 141) -> (junction 143) : {
          |  VDKC_CmdDelayDone_flg = TRUE;
          | }
      (junction 143) -> (junction 142)
      (junction 144) -> (junction 143)
    state UWDLock_Cmd_Delay
      (default) -> (junction 30) : {
          |  VDKC_CmdDelayTime_s = 0;
          |  VDKC_CmdDelayDone_flg = FALSE;
          | }
      UWDLock_Cmd_Delay -> (junction 30) [order 1]
      (junction 30) -> (junction 35) [order 1] : [ VDKC_CmdDelayTime_s > KDKC_LockCmdDelayTime_s]
      (junction 30) -> (junction 33) [order 2]
      (junction 35) -> (junction 106) : {
          |  VDKC_CmdDelayDone_flg = TRUE;
          | }
      (junction 33) -> (junction 109) [order 1] : [ VDKC_PCmdFallingEdge_flg == TRUE]
      (junction 33) -> (junction 105) [order 2] : {
          |  VDKC_CmdDelayTime_s += task_time_s;
          | }
      (junction 109) -> (junction 107) : {
          |  VDKC_CmdDelayDone_flg = TRUE;
          | }
      (junction 107) -> (junction 105)
      (junction 106) -> (junction 107)
    state UWBUnlock_Cmd_Delay
      (default) -> (junction 47) : {
          |  VDKC_CmdDelayTime_s = 0;
          |  VDKC_CmdDelayDone_flg = FALSE;
          | }
      UWBUnlock_Cmd_Delay -> (junction 47) [order 1]
      (junction 47) -> (junction 45) [order 1] : [ VDKC_CmdDelayTime_s > KDKC_UnlockCmdDelayTime_s]
      (junction 47) -> (junction 53) [order 2]
      (junction 45) -> (junction 117) : {
          |  VDKC_CmdDelayDone_flg = TRUE;
          | }
      (junction 53) -> (junction 118) [order 1] : [ VDKC_PCmdFallingEdge_flg == TRUE]
      (junction 53) -> (junction 115) [order 2] : {
          |  VDKC_CmdDelayTime_s += task_time_s;
          | }
      (junction 118) -> (junction 116) : {
          |  VDKC_CmdDelayDone_flg = TRUE;
          | }
      (junction 116) -> (junction 115)
      (junction 117) -> (junction 116)
    state UWB_DKC_Cmd_Default
      en:
      VDKC_CmdHandling_flg = FALSE;
      VDKC_UWBPCmdToBCMRAW_enum = ENUM_PCMDTOBCM_DEFAULT;
      VDKC_UWBPCmdHandingSta_enum=ENUM_DKCPCMDHANDING_OVER;%ENUM_UWBPCmdHanding_over
    (default) -> (junction 5) : {VDKC_CmdHandling_flg = FALSE;}
    UWB -> (junction 5) : [ !VDKC_CmdHandling_flg ]
    (junction 5) -> (junction 10) [order 2]
    (junction 5) -> (junction 8) [order 1] : [ VPMM_PowerSta_enum != ENUM_POWERSTA_READY]
    (junction 10) -> UWB_DKC_Cmd_Default
    (junction 8) -> (junction 97) [order 1] : [ VDKC_UWBDetReqtoUnlock_flg == TRUE]
    (junction 97) -> (junction 14) [order 1] : [ VBCM_AntitheftSta_enum ==ENUM_ANTITHEFT_ALARM ||...
        |   VBCM_AntitheftSta_enum == ENUM_ANTITHEFT_ARM]
    (junction 8) -> (junction 84) [order 2]
    (junction 97) -> UWB_DKC_Cmd_Default [order 2]
    (junction 14) -> UWBUnlock_Cmd_Delay : {
        | VDKC_CmdHandling_flg = TRUE;
        | VDKC_UWBPCmdToBCMRAW_enum = ENUM_PCMDTOBCM_UWBUNLOCK;
        | VDKC_UWBPCmdHandingSta_enum =ENUM_DKCPCMDHANDING_UNLOCK;
        | }
    (junction 84) -> (junction 87) [order 1] : [ VDKC_UWBDetReqtoLock_flg == TRUE]
    (junction 84) -> (junction 170) [order 2]
    (junction 87) -> (junction 91)
    (junction 170) -> (junction 172) [order 1] : [ VINP_SeatSW_flg==FALSE ]
    (junction 170) -> UWB_DKC_Cmd_Default [order 2]
    (junction 172) -> (junction 183)
    (junction 91) -> (junction 90) [order 1] : [ VBCM_AntitheftSta_enum ==ENUM_ANTITHEFT_DISARM ||...
        |   VBCM_AntitheftSta_enum == ENUM_ANTITHEFT_WAIT]
    (junction 91) -> UWB_DKC_Cmd_Default [order 2]
    (junction 90) -> UWDLock_Cmd_Delay : {
        | VDKC_CmdHandling_flg = TRUE;
        | VDKC_UWBPCmdToBCMRAW_enum = ENUM_PCMDTOBCM_UWBLOCK;
        | VDKC_UWBPCmdHandingSta_enum =ENUM_DKCPCMDHANDING_LOCK;
        | }
    (junction 183) -> (junction 184) [order 1] : [ VDKC_UIDDetRSSIChgToLock_flg==TRUE&&VPMM_PowerSta_enum != ENUM_POWERSTA_ON ]
    (junction 183) -> (junction 191) [order 2]
    (junction 184) -> (junction 159)
    (junction 191) -> (junction 193) [order 1] : [VDKC_UnavToUnlReqUnlock_flg==TRUE]
    (junction 191) -> UWB_DKC_Cmd_Default [order 2]
    (junction 193) -> (junction 215)
    (junction 159) -> (junction 163) [order 1] : [ VBCM_AntitheftSta_enum ==ENUM_ANTITHEFT_DISARM ||...
        |   VBCM_AntitheftSta_enum == ENUM_ANTITHEFT_WAIT]
    (junction 215) -> (junction 217) [order 1] : [ VBCM_AntitheftSta_enum ==ENUM_ANTITHEFT_ALARM ||...
        |   VBCM_AntitheftSta_enum == ENUM_ANTITHEFT_ARM]
    (junction 215) -> UWB_DKC_Cmd_Default [order 2]
    (junction 159) -> UWB_DKC_Cmd_Default [order 2]
    (junction 163) -> RSSILock_Cmd_Delay : {
        | VDKC_CmdHandling_flg = TRUE;
        | VDKC_UWBPCmdToBCMRAW_enum = ENUM_PCMDTOBCM_UWBLOCK;
        | VDKC_UWBPCmdHandingSta_enum =ENUM_DKCPCMDHANDING_LOCK;
        | }
    (junction 217) -> UnavToUnLockReqUnlock_Cmd_Delay : {
        | VDKC_CmdHandling_flg = TRUE;
        | VDKC_UWBPCmdToBCMRAW_enum = ENUM_PCMDTOBCM_UWBUNLOCK;
        | VDKC_UWBPCmdHandingSta_enum =ENUM_DKCPCMDHANDING_UNLOCK;
        | }
    UnavToUnLockReqUnlock_Cmd_Delay -> UWB_DKC_Cmd_Default [order 1] : [ VDKC_CmdDelayDone_flg ]
    RSSILock_Cmd_Delay -> UWB_DKC_Cmd_Default [order 1] : [ VDKC_CmdDelayDone_flg ]
    UWDLock_Cmd_Delay -> UWB_DKC_Cmd_Default [order 1] : [ VDKC_CmdDelayDone_flg ]
    UWBUnlock_Cmd_Delay -> UWB_DKC_Cmd_Default [order 1] : [ VDKC_CmdDelayDone_flg ]
  data: KDKC_LockCmdDelayTime_s input single; KDKC_UnlockCmdDelayTime_s input single; VBCM_AntitheftSta_enum input uint8; VDKC_UWBDetReqtoLock_flg input boolean; VDKC_UWBDetReqtoUnlock_flg input boolean; VDKC_UIDDetRSSIChgToLock_flg input boolean; VDKC_UnavToUnlReqUnlock_flg input boolean; task_time_s input single; VDKC_CmdHandling_flg local boolean; VDKC_CmdDelayTime_s local single; ENUM_ANTITHEFT_ALARM parameter; ENUM_ANTITHEFT_ARM parameter; ENUM_PCMDTOBCM_DEFAULT parameter; FALSE parameter; TRUE parameter; VDKC_UWBPCmdToBCMRAW_enum output uint8; ENUM_POWERSTA_READY parameter; VPMM_PowerSta_enum input uint8; VINP_SeatSW_flg input boolean; VDKC_UWBPCmdHandingSta_enum output uint8; ENUM_ANTITHEFT_DISARM parameter; ENUM_ANTITHEFT_WAIT parameter; ENUM_DKCPCMDHANDING_LOCK parameter; ENUM_DKCPCMDHANDING_UNLOCK parameter; ENUM_DKCPCMDHANDING_OVER parameter; VDKC_PCmdFallingEdge_flg input boolean; VDKC_CmdDelayDone_flg local boolean; ENUM_PCMDTOBCM_UWBLOCK parameter; ENUM_PCMDTOBCM_UWBUNLOCK parameter; ENUM_POWERSTA_ON parameter

== stateflow chart dkc/DKC/Subsystem/DKC_Handler/PDkeyJudgeBatLowVolt_Chart ==
  state PDkeyJudgeBatLowVolt_Chart
    (default) -> (junction 119) : {
        |  VDKC_UIDBatLowVolt_flg=0;
        |  VDKC_VoltCheckMode=0;
        |  SampTimeCounter=0;
        |  UIDBatSamp_cnt=0;
        |  UIDBatOKVolDet_Cnt=0;
        |  UIDBatLowVolDet_Cnt=0;
        | }
    PDkeyJudgeBatLowVolt_Chart -> (junction 119)
    (junction 119) -> (junction 121) [order 1] : [VDKC_BTConnectSta_enum==ENUM_BTCONNSTA_CONNECTED]
    (junction 119) -> (junction 127) [order 2] : {
        |  VDKC_UIDBatLowVolt_flg=0;
        |  VDKC_VoltCheckMode=0;
        |  SampTimeCounter=0;
        |  UIDBatSamp_cnt=0;
        |  UIDBatOKVolDet_Cnt=0;
        |  UIDBatLowVolDet_Cnt=0;
        | }
    (junction 121) -> (junction 4) : {
        |
        | SampTimeCounter = SampTimeCounter + 1;
        | }
    (junction 4) -> (junction 9) [order 1] : [SampTimeCounter>=(KDKC_UIDBatSampInterval_s/task_time_s)]
    (junction 4) -> (junction 11) [order 2]
    (junction 9) -> (junction 65) : {
        | SampTimeCounter=0;
        | }
    (junction 65) -> (junction 67) [order 1] : [UIDBatSamp_cnt>=KDKC_UIDBatSampTotal_cnt]
    (junction 65) -> (junction 91) [order 2] : {
        | UIDBatSamp_cnt = UIDBatSamp_cnt + 1;
        | }
    (junction 67) -> (junction 13) : {UIDBatSamp_cnt=0;}
    (junction 91) -> (junction 89) [order 1] : [VDKC_VoltCheckMode==0]%UIDLowBat Check mode
    (junction 13) -> (junction 23) [order 1] : [VDKC_VoltCheckMode==0]%UIDLowBat Check mode
    (junction 91) -> (junction 77) [order 2] : %UIDBatty OK Check mode
    (junction 89) -> (junction 93)
    (junction 13) -> (junction 101) [order 2] : %UIDBatty OK Check mode
    (junction 23) -> (junction 31)
    (junction 77) -> (junction 75) [order 1] : [VDKC_UIDBatVoltx1000_V>KDKC_UIDBatOKVolx1000Thres_V]
    (junction 93) -> (junction 84) [order 1] : [VDKC_UIDBatVoltx1000_V<KDKC_UIDBatLowVolx1000Thres_V]
    (junction 101) -> (junction 97) [order 1] : [UIDBatOKVolDet_Cnt>=KDKC_UIDBatOKVolDeb_cnt]
    (junction 31) -> (junction 35) [order 1] : [UIDBatLowVolDet_Cnt>=KDKC_UIDBatLowVolDeb_cnt]
    (junction 77) -> (junction 74) [order 2]
    (junction 75) -> (junction 73) : {UIDBatOKVolDet_Cnt = UIDBatOKVolDet_Cnt + 1;
        | }
    (junction 93) -> (junction 83) [order 2]
    (junction 84) -> (junction 81) : {UIDBatLowVolDet_Cnt = UIDBatLowVolDet_Cnt + 1;
        | }
    (junction 101) -> (junction 98) [order 2] : {VDKC_UIDBatLowVolt_flg=1;%output flg
        | VDKC_VoltCheckMode=1;%keep OKVol Check Mode
        | }
    (junction 97) -> (junction 96) : {VDKC_UIDBatLowVolt_flg=0;%output flg
        |  VDKC_VoltCheckMode=0;%Switch LowVol Check Mode
        | }
    (junction 31) -> (junction 37) [order 2] : {VDKC_UIDBatLowVolt_flg=0;%output flg
        | VDKC_VoltCheckMode=0;%keep LowVol Check Mode
        | }
    (junction 35) -> (junction 50) : {VDKC_UIDBatLowVolt_flg=1;%output flg
        |  VDKC_VoltCheckMode=1;%Switch OK Vol CheckMode
        | }
    (junction 73) -> (junction 74)
    (junction 81) -> (junction 83)
    (junction 96) -> (junction 98)
    (junction 50) -> (junction 37)
    (junction 74) -> (junction 111)
    (junction 83) -> (junction 109)
    (junction 98) -> (junction 106) : {UIDBatOKVolDet_Cnt=0;
        | UIDBatLowVolDet_Cnt=0;}
    (junction 37) -> (junction 104) : {UIDBatOKVolDet_Cnt=0;
        | UIDBatLowVolDet_Cnt=0;}
    (junction 11) -> (junction 127)
    (junction 111) -> (junction 11)
    (junction 109) -> (junction 111)
    (junction 106) -> (junction 109)
    (junction 104) -> (junction 106)
  data: VDKC_UIDBatVoltx1000_V input; KDKC_UIDBatLowVolx1000Thres_V input; KDKC_UIDBatOKVolx1000Thres_V input; VDKC_VoltCheckMode local uint8; KDKC_UIDBatLowVolDeb_cnt input; KDKC_UIDBatOKVolDeb_cnt input; KDKC_UIDBatSampInterval_s input; KDKC_UIDBatSampTotal_cnt input; VDKC_BTConnectSta_enum input; task_time_s input; UIDBatSamp_cnt local uint16; UIDBatLowVolDet_Cnt local uint16; SampTimeCounter local single; UIDBatOKVolDet_Cnt local uint16; ENUM_BTCONNSTA_CONNECTED parameter; VDKC_UIDBatLowVolt_flg output boolean

== stateflow chart dkc/DKC/Subsystem/DKC_Handler/TrunkHanSW_PCMD_Chart ==
  state TrunkHanSW_PCMD_Chart
    state TrunkHanSWUnlock_Cmd_Delay
      (default) -> (junction 30) : {
          |  VDKC_CmdDelayTime_s = 0;
          |  VDKC_CmdDelayDone_flg = FALSE;
          | }
      TrunkHanSWUnlock_Cmd_Delay -> (junction 30) [order 1]
      (junction 30) -> (junction 35) [order 1] : [ VDKC_CmdDelayTime_s > KDKC_UnlockCmdDelayTime_s]
      (junction 30) -> (junction 33) [order 2]
      (junction 35) -> (junction 106) : {
          |  VDKC_CmdDelayDone_flg = TRUE;
          | }
      (junction 33) -> (junction 109) [order 1] : [ VDKC_PCmdFallingEdge_flg == TRUE]
      (junction 33) -> (junction 105) [order 2] : {
          |  VDKC_CmdDelayTime_s += task_time_s;
          | }
      (junction 109) -> (junction 107) : {
          |  VDKC_CmdDelayDone_flg = TRUE;
          | }
      (junction 107) -> (junction 105)
      (junction 106) -> (junction 107)
    state TrunkHanUnlock_Cmd_Default
      en:
      VDKC_CmdHandling_flg = FALSE;
      VDKC_TrunkHanPCmdToBCMRAW_enum = ENUM_PCMDTOBCM_DEFAULT;
      VDKC_TrunkHanUnlockPCmdHandingSta_enum=ENUM_DKCPCMDHANDING_OVER;
    (default) -> (junction 5) : {VDKC_CmdHandling_flg = FALSE;}
    TrunkHanSW_PCMD_Chart -> (junction 5) : [ !VDKC_CmdHandling_flg ]
    (junction 5) -> (junction 10) [order 2]
    (junction 5) -> (junction 84) [order 1] : [VDKC_VehSpeed_kph<=0&&....
        |   (VDKC_GearActualPosn_enum==ENUM_GEARACTUALPOSN_P||....
        |    VDKC_GearActualPosn_enum==ENUM_GEARACTUALPOSN_N)]
    (junction 10) -> TrunkHanUnlock_Cmd_Default
    (junction 84) -> (junction 87) [order 1] : [ VDKC_TrunkHanSW_flg == TRUE]
    (junction 84) -> TrunkHanUnlock_Cmd_Default [order 2]
    (junction 87) -> (junction 91)
    (junction 91) -> (junction 90) [order 1] : [ VBCM_AntitheftSta_enum ==ENUM_ANTITHEFT_ARM ||...
        |   VBCM_AntitheftSta_enum == ENUM_ANTITHEFT_ALARM]
    (junction 91) -> TrunkHanUnlock_Cmd_Default [order 2]
    (junction 90) -> TrunkHanSWUnlock_Cmd_Delay : {
        | VDKC_CmdHandling_flg = TRUE;
        | VDKC_TrunkHanPCmdToBCMRAW_enum = ENUM_PCMDTOBCM_TGATEHANDLE;
        | VDKC_TrunkHanUnlockPCmdHandingSta_enum =ENUM_DKCPCMDHANDING_TGATEHANDLE;
        | }
    TrunkHanSWUnlock_Cmd_Delay -> TrunkHanUnlock_Cmd_Default [order 1] : [ VDKC_CmdDelayDone_flg ]
  data: KDKC_UnlockCmdDelayTime_s input single; VBCM_AntitheftSta_enum input uint8; VDKC_TrunkHanSW_flg input boolean; task_time_s input single; VDKC_CmdHandling_flg local boolean; ENUM_PCMDTOBCM_DEFAULT parameter; FALSE parameter; TRUE parameter; ENUM_DKCPCMDHANDING_OVER parameter; VDKC_PCmdFallingEdge_flg input boolean; VDKC_VehSpeed_kph input; VDKC_CmdDelayDone_flg local boolean; VDKC_CmdDelayTime_s local single; ENUM_ANTITHEFT_ARM parameter; ENUM_ANTITHEFT_ALARM parameter; VDKC_TrunkHanPCmdToBCMRAW_enum output uint8; VDKC_TrunkHanUnlockPCmdHandingSta_enum output uint8; ENUM_DKCPCMDHANDING_TGATEHANDLE parameter; ENUM_PCMDTOBCM_TGATEHANDLE parameter; ENUM_GEARACTUALPOSN_N parameter; ENUM_GEARACTUALPOSN_P parameter; VDKC_GearActualPosn_enum input

== stateflow chart dkc/DKC/Subsystem/DKC_Scheduler ==
  state trigger_100ms
    (default) -> (junction 1) : {
        | counter = 0;
        | }
    trigger_100ms -> (junction 1) : {
        | counter++;
        | }
    (junction 1) -> (junction 8) [order 1] : [counter%%uint8((0.1/task_time_s)) == 0]  /* 100ms trigger */
    (junction 1) -> (junction 5) [order 2]
    (junction 8) -> (junction 9) : {
        | trig_DKCcounter_100ms;
        | counter = 0;
        | }
    (junction 9) -> (junction 5)
  data: counter local uint32 size=1; task_time_s input
  events: trig_DKCcounter_100ms output FUNCTION_CALL_EVENT
